simulink model "sampleModel1533_2_sub_sub_sub"  (R2023a)
settings: Solver=VariableStepAuto  StartTime=0.0  StopTime=10.0  RelTol=1e-3
libraries: hdlsllib x2, simulink x1
settings Model: Creator=user1  LastModifiedBy=user1

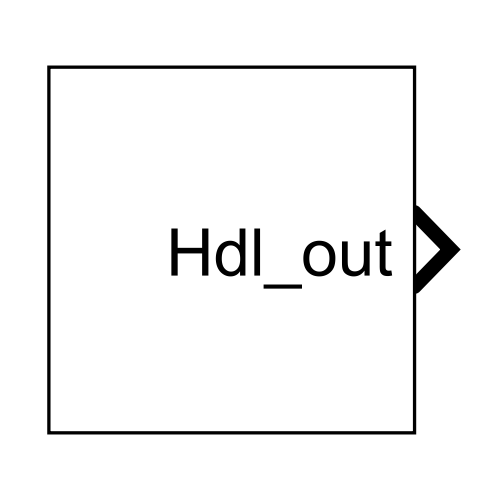
[thumbnail: Simulink's stored preview of the top-level diagram]
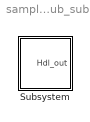
== system sampleModel1533_2_sub_sub_sub ==
  Subsystem : Subsystem

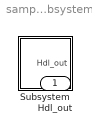
== system sampleModel1533_2_sub_sub_sub/Subsystem ==
  Subsystem : Subsystem
  Hdl_out : Outport  OutDataTypeStr=uint8

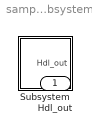
== system sampleModel1533_2_sub_sub_sub/Subsystem/Subsystem ==
  Subsystem : Subsystem
  Hdl_out : Outport  OutDataTypeStr=uint8

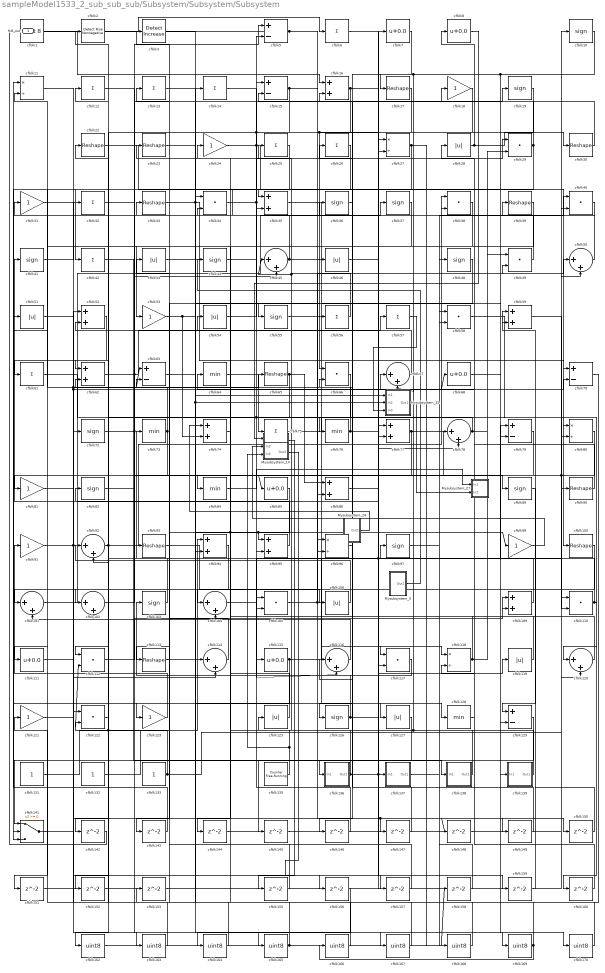
== system sampleModel1533_2_sub_sub_sub/Subsystem/Subsystem/Subsystem ==
  Mysubsystem_14 : Subsystem  TreatAsAtomicUnit=on  RTWFcnName=Mysubsystem_14
      settings: RTWFcnNameOpts=User specified  RTWFileNameOpts=Use function name
  Mysubsystem_24 : Subsystem  TreatAsAtomicUnit=on  RTWFcnName=Mysubsystem_24
      settings: RTWFcnNameOpts=User specified  RTWFileNameOpts=Use function name
  Mysubsystem_27 : Subsystem  TreatAsAtomicUnit=on  RTWFcnName=Mysubsystem_27
      settings: RTWFcnNameOpts=User specified  RTWFileNameOpts=Use function name
  Mysubsystem_31 : Subsystem  TreatAsAtomicUnit=on  RTWFcnName=Mysubsystem_31
      settings: RTWFcnNameOpts=User specified  RTWFileNameOpts=Use function name
  Mysubsystem_5 : Subsystem  TreatAsAtomicUnit=on  RTWFcnName=Mysubsystem_5
      settings: RTWFcnNameOpts=User specified  RTWFileNameOpts=Use function name
  cfblk1 : ArithShift  BitShiftNumber=8
  cfblk{10,19,36..37,41,44,48,55,72,82,89,97,103,126} (14 alike) : Signum
  cfblk{17,22..23,30,33,39,65,90,93,100,113} (11 alike) : Reshape
  cfblk{45,50,67,78,92,101..102,104,114,116,120} (11 alike) : Sum  Inputs=|++  OutDataTypeStr=uint8
  cfblk{29,34,38,40,49,58,66,105,110,112,117,122} (12 alike) : DotProduct  OutDataTypeStr=uint8
  cfblk{28,43,46,51,54,106,119,125,127} (9 alike) : Abs  OutDataTypeStr=uint8  SaturateOnIntegerOverflow=off
  cfblk{16,35,52,59,62,74,77,86,94..95,109} (11 alike) : Sum  OutDataTypeStr=uint8
  cfblk{11,27,80,96,118} (5 alike) : Product  Inputs=*/  OutDataTypeStr=uint8  RndMeth=Zero  SaturateOnIntegerOverflow=on
  cfblk{7..8,68,85,111,115} (6 alike) : Bias  Bias=0.0  SaturateOnIntegerOverflow=off
  cfblk{6,12..14,25..26,32,42,56..57,61,75} (12 alike) : Sum  Inputs=+  OutDataTypeStr=uint8
  cfblk{18,24,31,53,81,91,99,121,123} (9 alike) : Gain  OutDataTypeStr=uint8
  cfblk{64,73,76,84,128} (5 alike) : MinMax  OutDataTypeStr=uint8
  cfblk{5,15,63,70,79,129} (6 alike) : Sum  Inputs=+-  OutDataTypeStr=uint8
  cfblk131 : Constant  OutDataTypeStr=uint8  SampleTime=-1
  cfblk132 : Constant  OutDataTypeStr=uint8  SampleTime=-1
  cfblk133 : Constant  OutDataTypeStr=uint8  SampleTime=-1
  cfblk135 : hdlsllib/Sources/Counter Free-Running  NumBits=16  tsamp=-1
  cfblk136 : Subsystem
      settings: LibrarySourceBlock=|
      | hdlsllib/Ports &
      | Subsystems/Subsystem
  cfblk137 : Subsystem
      settings: LibrarySourceBlock=|
      | hdlsllib/Ports &
      | Subsystems/Subsystem
  cfblk138 : Subsystem
      settings: LibrarySourceBlock=|
      | hdlsllib/Ports &
      | Subsystems/Subsystem
  cfblk139 : Subsystem
      settings: LibrarySourceBlock=|
      | hdlsllib/Ports &
      | Subsystems/Subsystem
  cfblk141 : Switch  OutDataTypeStr=uint8  SaturateOnIntegerOverflow=off  InputSameDT=off
  cfblk{142..153,155..160} (18 alike) : Delay  SampleTime=1
  cfblk{162..170} (9 alike) : DataTypeConversion  OutDataTypeStr=uint8  SaturateOnIntegerOverflow=off  RndMeth=Floor
  cfblk2 : hdlsllib/Logic and Bit Operations/Detect Rise Nonnegative  vinit=0  OutDataTypeStr=uint8
  cfblk3 : simulink/Logic and Bit Operations/Detect Increase  vinit=0.0  OutDataTypeStr=uint8
      settings: LibrarySourceBlock=|
      | hdlsllib/Logic and Bit
      | Operations/Detect
      | Increase
  Hdl_out : Outport  OutDataTypeStr=uint8
  wires:
  cfblk118/1 -> cfblk49/1, cfblk33/1
  cfblk55/1 -> cfblk117/1
  cfblk26/1 -> cfblk35/1
  cfblk1/1 -> cfblk16/1
  cfblk90/1 -> cfblk64/1
  cfblk117/1 -> cfblk103/1
  cfblk45/1 -> cfblk31/1, cfblk128/1
  cfblk42/1 -> cfblk138/1(In1)
  cfblk40/1 -> cfblk42/1
  cfblk73/1 -> cfblk142/1, cfblk11/2
  cfblk28/1 -> cfblk8/1, cfblk30/1
  cfblk131/1 -> cfblk14/1
  cfblk91/1 -> cfblk157/1, cfblk37/1
  cfblk80/1 -> cfblk110/2, cfblk85/1
  cfblk18/1 -> cfblk62/1, cfblk66/1
  cfblk58/1 -> cfblk120/1
  cfblk63/1 -> cfblk95/1, cfblk99/1
  cfblk128/1 -> cfblk28/1
  cfblk2/1 -> cfblk6/1
  cfblk3/1 -> cfblk169/1
  cfblk62/1 -> cfblk86/2, cfblk57/1
  cfblk110/1 -> cfblk160/1, cfblk22/1
  cfblk22/1 -> cfblk100/1
  cfblk33/1 -> cfblk55/1, Mysubsystem_31/1(In1)
  cfblk46/1 -> cfblk27/1
  cfblk95/1 -> cfblk41/1
  cfblk24/1 -> cfblk106/1, cfblk96/1
  cfblk27/1 -> cfblk168/1, cfblk146/1
  cfblk43/1 -> cfblk96/2
  cfblk53/1 -> cfblk74/2, cfblk89/1, Mysubsystem_31/2(In2)
  cfblk104/1 -> cfblk97/1
  cfblk94/1 -> cfblk113/1
  cfblk114/1 -> cfblk13/1
  cfblk39/1 -> cfblk53/1
  cfblk132/1 -> cfblk94/1
  cfblk5/1 -> Hdl_out/1, cfblk148/1, cfblk147/1
  cfblk77/1 -> cfblk102/2, cfblk139/1(In1)
  cfblk120/1 -> cfblk59/1
  cfblk13/1 -> cfblk56/1
  cfblk19/1 -> cfblk35/2
  cfblk103/1 -> cfblk73/1
  cfblk123/1 -> cfblk91/1
  cfblk75/1 -> cfblk80/1
  cfblk92/1 -> cfblk152/1, cfblk38/1
  cfblk138/1(Out1) -> cfblk125/1
  cfblk93/1 -> cfblk105/2
  cfblk105/1 -> cfblk49/2, cfblk10/1
  cfblk115/1 -> cfblk141/3, cfblk77/2, cfblk79/1
  cfblk41/1 -> cfblk32/1
  cfblk126/1 -> cfblk70/2, cfblk43/1
  cfblk52/1 -> cfblk61/1
  cfblk64/1 -> cfblk75/1
  cfblk7/1 -> cfblk17/1
  cfblk102/1 -> cfblk19/1
  cfblk136/1(Out1) -> cfblk25/1, cfblk45/1, cfblk159/1, cfblk119/1
  cfblk109/1 -> cfblk2/1
  cfblk15/1 -> cfblk92/2, cfblk27/2
  cfblk97/1 -> cfblk48/1
  cfblk119/1 -> cfblk66/2
  cfblk59/1 -> cfblk90/1
  cfblk37/1 -> cfblk101/1
  cfblk54/1 -> cfblk15/1
  cfblk50/1 -> cfblk39/1
  cfblk16/1 -> cfblk78/2, cfblk95/2, cfblk112/1
  cfblk78/1 -> cfblk29/2, cfblk76/1
  cfblk111/1 -> cfblk63/1, cfblk52/1
  cfblk74/1 -> cfblk24/1
  cfblk67/1 -> cfblk54/1
  cfblk137/1(Out1) -> cfblk40/1
  cfblk81/1 -> cfblk68/1, cfblk65/1
  cfblk85/1 -> cfblk144/1, cfblk143/1
  cfblk35/1 -> cfblk79/2
  cfblk30/1 -> cfblk15/2
  cfblk36/1 -> cfblk126/1
  cfblk113/1 -> cfblk114/1
  cfblk29/1 -> cfblk141/2, cfblk18/1
  cfblk127/1 -> cfblk141/1
  cfblk125/1 -> cfblk93/1
  cfblk133/1 -> cfblk50/2, cfblk62/2, cfblk112/2
  cfblk89/1 -> cfblk129/1
  cfblk141/1 -> cfblk72/1
  cfblk25/1 -> cfblk81/1
  cfblk76/1 -> cfblk51/1, cfblk7/1
  cfblk14/1 -> cfblk70/1
  cfblk23/1 -> cfblk127/1
  cfblk65/1 -> cfblk86/1, cfblk104/1
  cfblk82/1 -> cfblk165/1
  cfblk56/1 -> cfblk23/1
  cfblk72/1 -> cfblk149/1, cfblk5/1
  cfblk86/1 -> cfblk50/1
  cfblk112/1 -> cfblk109/1
  cfblk44/1 -> cfblk29/1
  cfblk12/1 -> cfblk45/2
  cfblk31/1 -> cfblk114/2
  cfblk135/1 -> cfblk52/2, Mysubsystem_14/3(In3)
  cfblk6/1 -> cfblk118/1
  cfblk139/1(Out1) -> cfblk36/1, cfblk67/1
  cfblk49/1 -> cfblk38/2
  cfblk38/1 -> cfblk84/1
  cfblk17/1 -> cfblk94/2
  cfblk10/1 -> cfblk129/2, cfblk67/2, cfblk46/1
  cfblk100/1 -> cfblk111/1
  cfblk34/1 -> cfblk116/2, cfblk5/2
  cfblk101/1 -> cfblk78/1
  cfblk116/1 -> cfblk101/2
  cfblk32/1 -> cfblk136/1(In1)
  cfblk106/1 -> cfblk92/1
  cfblk96/1 -> cfblk26/1
  cfblk61/1 -> cfblk115/1, cfblk137/1(In1)
  cfblk48/1 -> cfblk123/1
  cfblk66/1 -> cfblk102/1
  cfblk142/1 -> cfblk1/1
  cfblk143/1 -> cfblk11/1
  cfblk144/1 -> cfblk120/2
  cfblk129/1 -> cfblk145/1
  cfblk145/1 -> cfblk80/2
  cfblk146/1 -> cfblk105/1
  cfblk147/1 -> cfblk16/2
  cfblk148/1 -> cfblk40/2
  cfblk149/1 -> cfblk116/1
  cfblk51/1 -> cfblk150/1
  cfblk150/1 -> cfblk59/2
  cfblk79/1 -> cfblk151/1
  cfblk151/1 -> cfblk117/2
  cfblk152/1 -> cfblk110/1
  cfblk70/1 -> cfblk153/1
  cfblk153/1 -> cfblk77/1
  cfblk155/1 -> cfblk63/2
  cfblk157/1 -> cfblk104/2
  cfblk158/1 -> cfblk58/1
  cfblk159/1 -> cfblk109/2
  cfblk160/1 -> cfblk118/2
  cfblk122/1 -> cfblk162/1
  cfblk162/1 -> cfblk58/2
  cfblk11/1 -> cfblk163/1
  cfblk163/1 -> cfblk122/1
  cfblk156/1 -> cfblk164/1
  cfblk164/1 -> cfblk122/2
  cfblk165/1 -> cfblk12/1, cfblk158/1
  cfblk166/1 -> cfblk82/1
  cfblk121/1 -> cfblk167/1
  cfblk167/1 -> cfblk34/1
  cfblk168/1 -> cfblk121/1
  cfblk169/1 -> cfblk34/2, cfblk166/1
  cfblk68/1 -> cfblk170/1
  cfblk170/1 -> cfblk3/1
  Mysubsystem_5/1(Out1) -> cfblk44/1
  cfblk8/1 -> Mysubsystem_14/1(In1)
  cfblk99/1 -> Mysubsystem_14/2(In2)
  Mysubsystem_14/1(Out1) -> cfblk155/1
  Mysubsystem_14/2(Out2) -> cfblk156/1
  Mysubsystem_24/1(Out1) -> cfblk74/1
  cfblk84/1 -> Mysubsystem_27/1(In1)
  cfblk57/1 -> Mysubsystem_31/3(In3)
  Mysubsystem_31/1(Out1) -> Mysubsystem_27/2(In2)

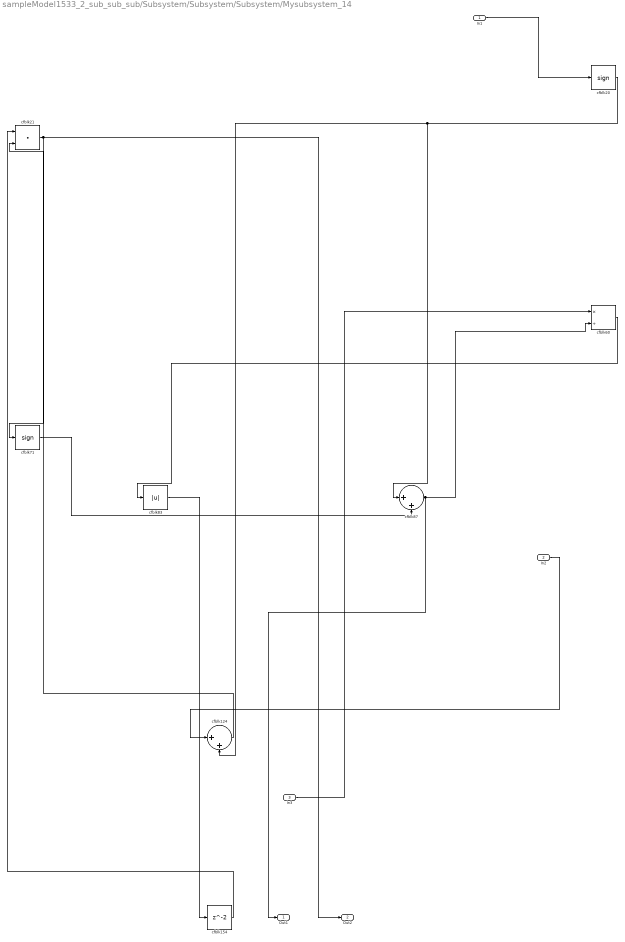
== system sampleModel1533_2_sub_sub_sub/Subsystem/Subsystem/Subsystem/Mysubsystem_14 ==
  In1 : Inport
  In2 : Inport  Port=2
  In3 : Inport  Port=3
  cfblk124 : Sum  Inputs=|++
  cfblk154 : Delay  SampleTime=1
  cfblk20 : Signum
  cfblk21 : DotProduct  OutDataTypeStr=Inherit: Inherit via internal rule
  cfblk60 : Product  Inputs=*/  RndMeth=Zero  SaturateOnIntegerOverflow=on
  cfblk71 : Signum
  cfblk83 : Abs  SaturateOnIntegerOverflow=off
  cfblk87 : Sum  Inputs=|++
  Out1 : Outport
  Out2 : Outport  Port=2
  wires:
  In1/1 -> cfblk20/1
  cfblk60/1 -> cfblk83/1
  cfblk87/1 -> cfblk60/2, Out1/1
  cfblk20/1 -> cfblk124/2, cfblk87/1
  cfblk124/1 -> cfblk21/2
  In2/1 -> cfblk124/1
  cfblk154/1 -> cfblk21/1
  cfblk21/1 -> cfblk71/1, Out2/1
  cfblk83/1 -> cfblk154/1
  In3/1 -> cfblk60/1
  cfblk71/1 -> cfblk87/2

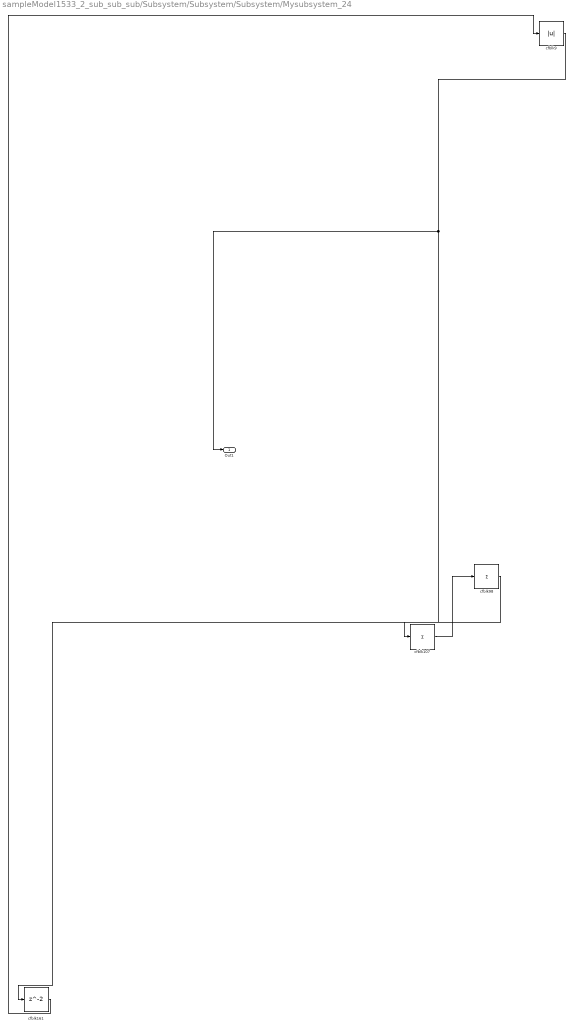
== system sampleModel1533_2_sub_sub_sub/Subsystem/Subsystem/Subsystem/Mysubsystem_24 ==
  cfblk107 : Sum  Inputs=+
  cfblk161 : Delay  SampleTime=1
  cfblk9 : Abs  SaturateOnIntegerOverflow=off
  cfblk98 : Sum  Inputs=+
  Out1 : Outport
  wires:
  cfblk161/1 -> cfblk9/1
  cfblk98/1 -> cfblk161/1
  cfblk9/1 -> cfblk107/1, Out1/1
  cfblk107/1 -> cfblk98/1

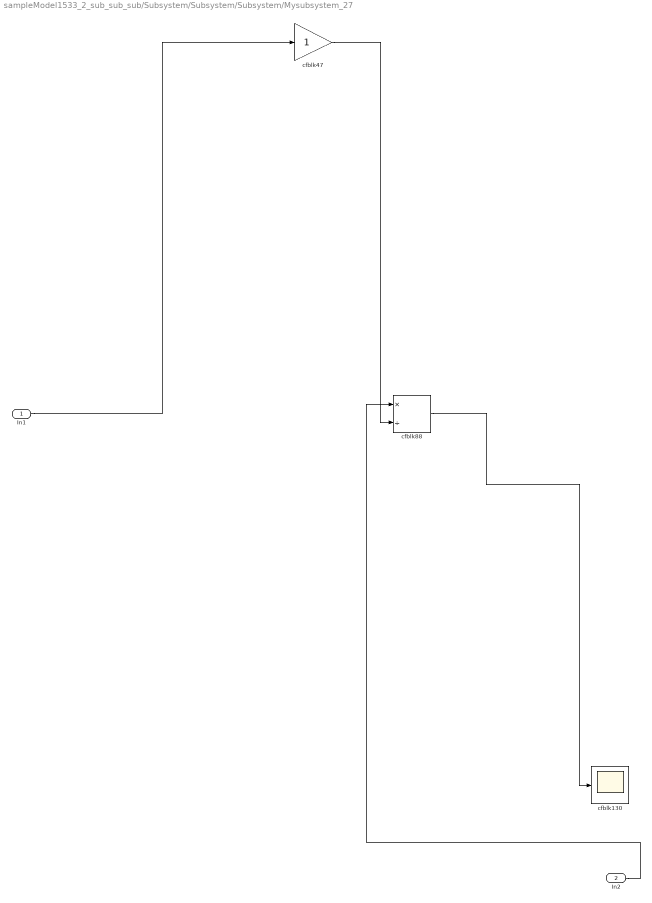
== system sampleModel1533_2_sub_sub_sub/Subsystem/Subsystem/Subsystem/Mysubsystem_27 ==
  In1 : Inport
  In2 : Inport  Port=2
  cfblk130 : Scope
  cfblk47 : Gain
  cfblk88 : Product  Inputs=*/  RndMeth=Zero  SaturateOnIntegerOverflow=on
  wires:
  In2/1 -> cfblk88/1
  In1/1 -> cfblk47/1
  cfblk88/1 -> cfblk130/1
  cfblk47/1 -> cfblk88/2

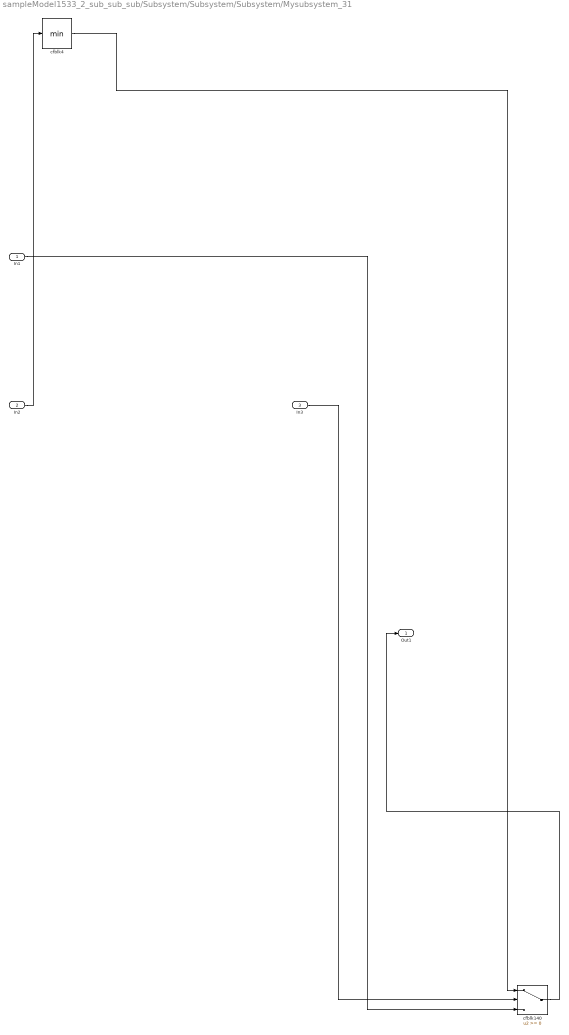
== system sampleModel1533_2_sub_sub_sub/Subsystem/Subsystem/Subsystem/Mysubsystem_31 ==
  In1 : Inport
  In2 : Inport  Port=2
  In3 : Inport  Port=3
  cfblk140 : Switch  SaturateOnIntegerOverflow=off  InputSameDT=off
  cfblk4 : MinMax
  Out1 : Outport
  wires:
  In2/1 -> cfblk4/1
  cfblk140/1 -> Out1/1
  In3/1 -> cfblk140/2
  In1/1 -> cfblk140/3
  cfblk4/1 -> cfblk140/1

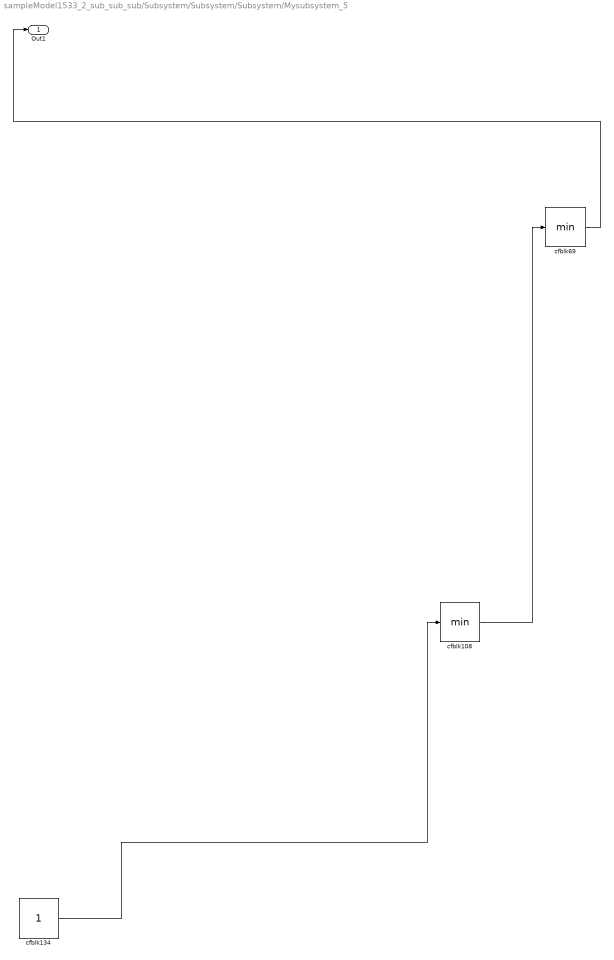
== system sampleModel1533_2_sub_sub_sub/Subsystem/Subsystem/Subsystem/Mysubsystem_5 ==
  cfblk108 : MinMax
  cfblk134 : Constant  SampleTime=-1
  cfblk69 : MinMax
  Out1 : Outport
  wires:
  cfblk69/1 -> Out1/1
  cfblk108/1 -> cfblk69/1
  cfblk134/1 -> cfblk108/1

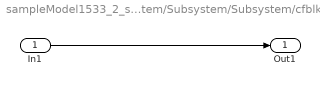
== system sampleModel1533_2_sub_sub_sub/Subsystem/Subsystem/Subsystem/cfblk136 ==
  In1 : Inport
  Out1 : Outport
  wires:
  In1/1 -> Out1/1

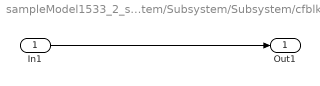
== system sampleModel1533_2_sub_sub_sub/Subsystem/Subsystem/Subsystem/cfblk137 ==
  In1 : Inport
  Out1 : Outport
  wires:
  In1/1 -> Out1/1

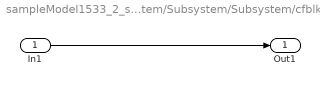
== system sampleModel1533_2_sub_sub_sub/Subsystem/Subsystem/Subsystem/cfblk138 ==
  In1 : Inport
  Out1 : Outport
  wires:
  In1/1 -> Out1/1

== system sampleModel1533_2_sub_sub_sub/Subsystem/Subsystem/Subsystem/cfblk139 ==
  In1 : Inport
  Out1 : Outport
  wires:
  In1/1 -> Out1/1
